simulink model "Plant_Model_HT_Cooling_Harness"  (R2022b)
settings: Solver=VariableStepAuto  StartTime=0.0  StopTime=60  RelTol=1e-3
settings Model: Creator=adrian.taveras  LastModifiedBy=stefan.notter

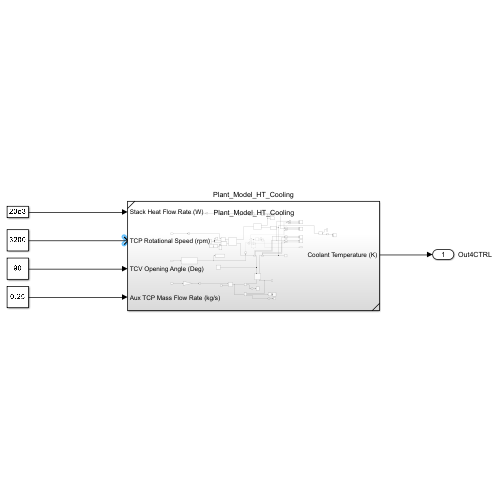
[thumbnail: Simulink's stored preview of the top-level diagram]
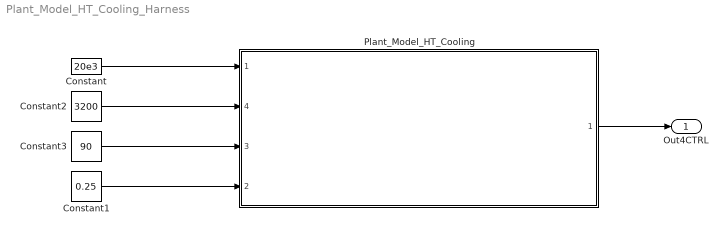
== system Plant_Model_HT_Cooling_Harness ==
  Constant : Constant  Value=20e3
  Constant1 : Constant  Value=0.25
  Constant2 : Constant  Value=3200
  Constant3 : Constant  Value=90
  Plant_Model_HT_Cooling : Subsystem  ReferencedSubsystem=Plant_Model_HT_Cooling
      settings: PortSchema="{\"entries\":[{\"content\":{\"sides\":[{\"content\":{\"connectorIds\":[\"Out1\"]},\"type\":\"ConnectorPlacement.EquallySpacedRectSide\",\"uuid\":\"706cf171-be05-45fb-992c-ba5e90f5cdb8\"},{\"content\":{\"connectorIds\":[\"In2\",\"In3\",\"In4\",\"In1\"],\"side\":\"RIGHT\"},\"type\":\"ConnectorPlacement.EquallySpacedRectSide\",\"uuid\":\"bf8ca14f-fef4-4eb5-a927-ccc799898aca\"},{\"content\":{\"connectorIds\":[],\"side\":\"TOP\"},\"type\":\"ConnectorPlacement.EquallySpacedRectSide\",\"uuid\":\"9ad70fe7-ae85-4ea7-9728-0856e6ff40bf\"}]},\"type\":\"ConnectorPlacement.EquallySpacedConnector\",\"uuid\":\"91c985a6-7405-42c3-ac14-8c35e74d3001\"}],\"packageUris\":[\"http://schema.mathworks.com/mf0/Connector/R2020b\"],\"version\":\"1.0\"}"
  Out4CTRL : Outport
  wires:
  Plant_Model_HT_Cooling/1 -> Out4CTRL/1
  Constant/1 -> Plant_Model_HT_Cooling/1
  Constant1/1 -> Plant_Model_HT_Cooling/2
  Constant2/1 -> Plant_Model_HT_Cooling/4
  Constant3/1 -> Plant_Model_HT_Cooling/3
